simulink model "UnitTest_Mavlink"  (R2020a)
settings: Solver=ode3  StartTime=0.0  StopTime=500  FixedStep=0.01  RelTol=1e-3
undefined symbols (not defined in the file or in its folder): MavlinkSimData
settings Model: Creator=Administrator  LastModifiedBy=Administrator

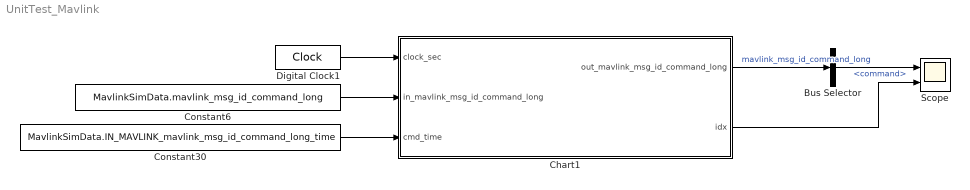
== system UnitTest_Mavlink ==
  Bus Selector : BusSelector  OutputSignals=command
  Chart1 : Stateflow chart  TreatAsAtomicUnit=on
  Constant30 : Constant  Value=MavlinkSimData.IN_MAVLINK_mavlink_msg_id_command_long_time
  Constant6 : Constant  Value=MavlinkSimData.mavlink_msg_id_command_long  OutDataTypeStr=Bus: mavlink_msg_id_command_long
  Digital Clock1 : DigitalClock  SampleTime=-1
  Scope : Scope  NumInputPorts=2
  wires:
  Constant30/1 -> Chart1/3(cmd_time)
  Constant6/1 -> Chart1/2(in_mavlink_msg_id_command_long)
  Digital Clock1/1 -> Chart1/1(clock_sec)
  Chart1/1(out_mavlink_msg_id_command_long) -> Bus Selector/1  "mavlink_msg_id_command_long"
  Bus Selector/1 -> Scope/1  "<command>"
  Chart1/2(idx) -> Scope/2

== stateflow chart UnitTest_Mavlink/Chart1 ==
  state Before
    en:
  state Doing
    en:
    idx = idx + 1;
    if in_mavlink_msg_id_command_long(idx).command ~= 0
    out_mavlink_msg_id_command_long = in_mavlink_msg_id_command_long(idx);
    end
    du:
  state After
    en:
    idx = idx + 1;
    if in_mavlink_msg_id_command_long(idx).command ~= 0
    out_mavlink_msg_id_command_long = in_mavlink_msg_id_command_long(idx);
    end
  (default) -> Before : {idx = 0;}
  Before -> Doing : [isOverFirstTime]
  (junction 20) -> Doing
  Doing -> (junction 15)
  (junction 15) -> (junction 20) [order 1] : [~isOverLastTime && isAllowGoToNext]
  (junction 15) -> After [order 2] : [isOverLastTime]
  data: flag function_output; flag function_output; flag function_output; clock_sec input; in_mavlink_msg_id_command_long input Bus: mavlink_msg_id_command_long size=200; out_mavlink_msg_id_command_long output Bus: mavlink_msg_id_command_long size=1; cmd_time input; idx output
  function flag = isOverLastTime:
    | function flag = isOverLastTime
    | flag = false;
    | if cmd_time(idx) == 0
    |     flag = true; 
    | end
  function flag = isOverFirstTime:
    | function flag = isOverFirstTime
    | % 达到第一个时间
    | flag = false;
    | if clock_sec >= cmd_time(1)
    |     flag = true; 
    | end
  function flag = isAllowGoToNext:
    | function flag = isAllowGoToNext
    | if idx < length(cmd_time) && ... % 索引保护
    |         cmd_time(idx+1) ~= 0     % 下一位为有效值
    |     time_threshold = cmd_time(idx+1);
    | else
    |     time_threshold = inf;
    | end
    | 
    | flag = false;
    | if clock_sec >= cmd_time(idx+1) && ...
    |         in_mavlink_msg_id_command_long(idx).command ~= 0
    |     flag = true; 
    | end
